simulink model "abc2dq"  (R2020a)
settings: Solver=VariableStepAuto  StartTime=0.0  StopTime=10.0  RelTol=1e-3
values from neighbouring files (symbols this model uses):
  Tss = 2.5e-6    (= 2.5e-06)    [parameters.m]
libraries: powerlib_meascontrol x2
settings Model: Creator=derek  LastModifiedBy=derek

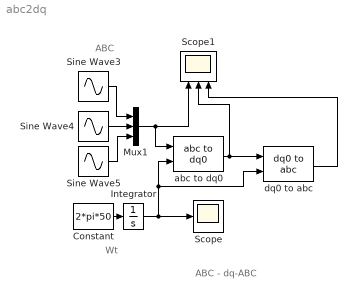
== system abc2dq ==
  note: ABC
  note: Wt
  note: ABC - dq-ABC
  Constant : Constant  Value=2*pi*50
  Integrator : Integrator
  Mux1 : Mux  Inputs=3
  Scope : Scope
  Scope1 : Scope  NumInputPorts=3
  Sine Wave3 : Sin  Amplitude=100  Frequency=2*pi*50  SampleTime=Tss
  Sine Wave4 : Sin  Amplitude=100  Frequency=2*pi*50  Phase=-((2*pi)/3)  SampleTime=Tss
  Sine Wave5 : Sin  Amplitude=100  Frequency=2*pi*50  Phase=((2*pi)/3)  SampleTime=Tss
  abc to dq0 : powerlib_meascontrol/Transformations/abc to dq0  Alignment=90 degrees behind phase A axis
  dq0 to abc : powerlib_meascontrol/Transformations/dq0 to abc  Alignment=90 degrees behind phase A axis
  wires:
  abc to dq0/1 -> dq0 to abc/1, Scope1/2
  Mux1/1 -> Scope1/1, abc to dq0/1
  Sine Wave4/1 -> Mux1/2
  Sine Wave5/1 -> Mux1/3
  Integrator/1 -> dq0 to abc/2, abc to dq0/2, Scope/1
  Sine Wave3/1 -> Mux1/1
  Constant/1 -> Integrator/1
  dq0 to abc/1 -> Scope1/3
